simulink model "simulation"  (R2023a)
settings: Solver=ode14x  StartTime=0.0  StopTime=75000.0  FixedStep=optimizerParams.simulinkStepSize  RelTol=1e-3
undefined symbols (not defined in the file or in its folder): ambientTemperatures, batteryParams, gridPricesDayBefore, optimizerParams, panelCurrentParams, panelTemperatureParams, powerDemand, solarIrradiation
libraries: simulink x4, dspsigops x4
settings Model: SimulationMode=accelerator  Creator=jespe  LastModifiedBy=jesperek
settings OptimizationCC: OptimizeBlockIOStorage=off  ReuseModelBlockBuffer=off
settings DebuggingCC: SignalResolutionControl=TryResolveAllWithWarning  SolverPrmCheckMsg=warning  UnderSpecifiedDataTypeMsg=warning  UnnecessaryDatatypeConvMsg=warning  VectorMatrixConversionMsg=warning  SignalLabelMismatchMsg=warning  UnconnectedInputMsg=warning  UnconnectedOutputMsg=warning  UnconnectedLineMsg=warning  SFcnCompatibilityMsg=warning  FrameProcessingCompatibilityMsg=warning  StateNameClashWarn=warning  StrictBusMsg=WarnOnBusTreatedAsVector  NonBusSignalsTreatedAsBus=warning  UnderSpecifiedDimensionMsg=warning
settings RTWCC: GenerateReport=on  BuildConfiguration=Debug  LaunchReport=on
settings CodeAppCC: ForceParamTrailComments=on  MaxIdLength=62  StateflowObjectComments=on  MATLABSourceComments=on

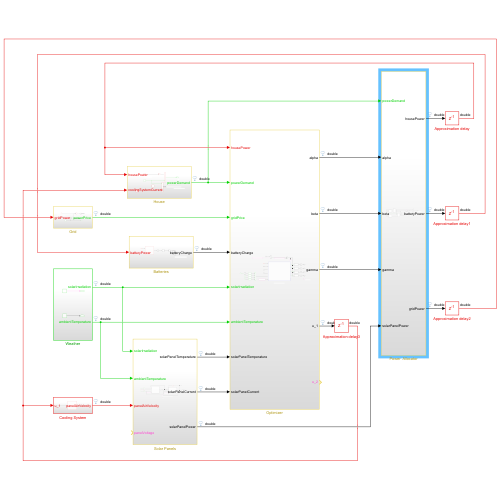
[thumbnail: Simulink's stored preview of the top-level diagram]
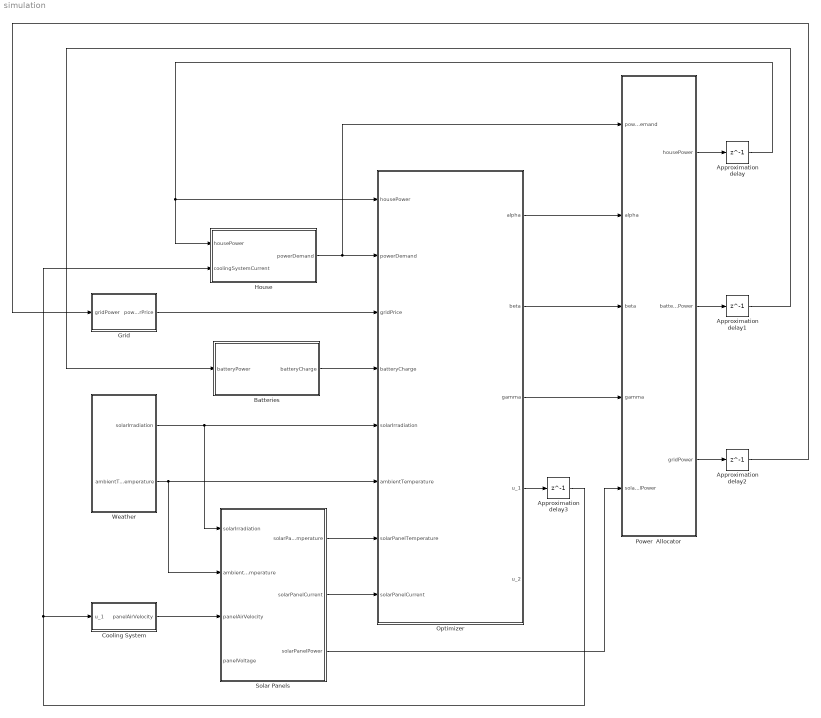
== system simulation ==
  Approximation delay{,1..3} (4 alike) : Delay  DelayLength=1  InitialCondition=0
  Batteries : Subsystem
  Cooling System : Subsystem
  Grid : Subsystem
  House : Subsystem
  Optimizer : Subsystem
  Power  Allocator : Subsystem
  Solar Panels : Subsystem
  Weather : Subsystem
  wires:
  Cooling System/1(panelAirVelocity) -> Solar Panels/3(panelAirVelocity)
  Weather/1(solarIrradiation) -> Solar Panels/1(solarIrradiation), Optimizer/5(solarIrradiation)
  Weather/2(ambientTemperature) -> Optimizer/6(ambientTemperature), Solar Panels/2(ambientTemperature)
  House/1(powerDemand) -> Power  Allocator/1(powerDemand), Optimizer/2(powerDemand)
  Grid/1(powerPrice) -> Optimizer/3(gridPrice)
  Solar Panels/3(solarPanelPower) -> Power  Allocator/5(solarPanelPower)
  Batteries/1(batteryCharge) -> Optimizer/4(batteryCharge)
  Power  Allocator/1(housePower) -> Approximation delay/1
  Power  Allocator/2(batteryPower) -> Approximation delay1/1
  Power  Allocator/3(gridPower) -> Approximation delay2/1
  Optimizer/1(alpha) -> Power  Allocator/2(alpha)
  Optimizer/2(beta) -> Power  Allocator/3(beta)
  Optimizer/3(gamma) -> Power  Allocator/4(gamma)
  Optimizer/4(u_1) -> Approximation delay3/1
  Solar Panels/2(solarPanelCurrent) -> Optimizer/8(solarPanelCurrent)
  Solar Panels/1(solarPanelTemperature) -> Optimizer/7(solarPanelTemperature)
  Approximation delay/1 -> Optimizer/1(housePower), House/1(housePower)
  Approximation delay1/1 -> Batteries/1(batteryPower)
  Approximation delay2/1 -> Grid/1(gridPower)
  Approximation delay3/1 -> Cooling System/1(u_1), House/2(coolingSystemCurrent)

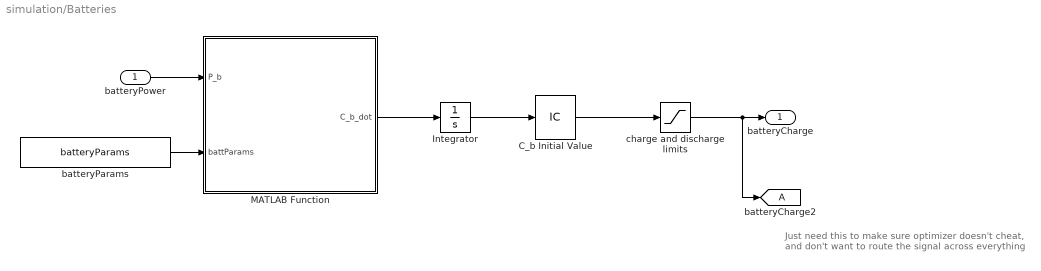
== system simulation/Batteries ==
  note: Just need this to make sure optimizer doesn't cheat,
      | and don't want to route the signal across everything
  batteryPower : Inport
  C_b Initial Value : InitialCondition  Value=0
  Integrator : Integrator
  MATLAB Function : MATLAB Function  TreatAsAtomicUnit=on
  batteryCharge2 : Goto  TagVisibility=global
  batteryParams : Constant  Value=batteryParams  OutDataTypeStr=Bus: battPars
  charge and discharge limits : Saturate  UpperLimit=batteryParams.maxCharge  LowerLimit=0.0
  batteryCharge : Outport
  wires:
  batteryPower/1 -> MATLAB Function/1(P_b)
  batteryParams/1 -> MATLAB Function/2(battParams)
  MATLAB Function/1(C_b_dot) -> Integrator/1
  Integrator/1 -> C_b Initial Value/1
  charge and discharge limits/1 -> batteryCharge/1, batteryCharge2/1
  C_b Initial Value/1 -> charge and discharge limits/1

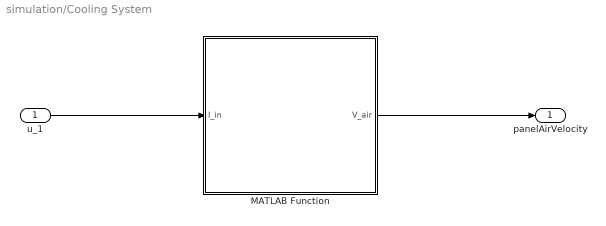
== system simulation/Cooling System ==
  u_1 : Inport
  MATLAB Function : MATLAB Function  TreatAsAtomicUnit=on
  panelAirVelocity : Outport
  wires:
  u_1/1 -> MATLAB Function/1(I_in)
  MATLAB Function/1(V_air) -> panelAirVelocity/1

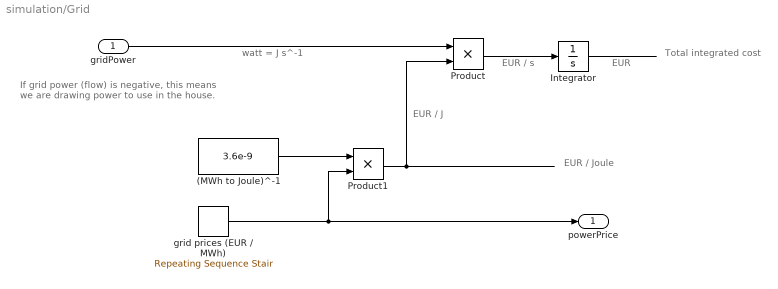
== system simulation/Grid ==
  note: EUR / J
  note: EUR
  note: EUR / s
  note: Total integrated cost
  note: watt = J s^-1
  note: If grid power (flow) is negative, this means
      | we are drawing power to use in the house.
  note: EUR / Joule
  gridPower : Inport
  (MWh to Joule)^-1 : Constant  Value=3.6e-9
  Integrator : Integrator
  Product : Product
  Product1 : Product
  grid prices (EUR / MWh) : simulink/Sources/Repeating Sequence Stair  OutValues=gridPrices  tsamp=1  OutMin=[]  OutMax=[]  OutDataTypeStr=double  OutputDataTypeScalingMode=double  OutDataType=fixdt(0,8)  ConRadixGroup=Best Precision: Vector-wise  OutScaling=2^-12
  powerPrice : Outport
  wires:
  gridPower/1 -> Product/1
  Product1/1 -> Product/2
  (MWh to Joule)^-1/1 -> Product1/1
  grid prices (EUR / MWh)/1 -> powerPrice/1, Product1/2
  Product/1 -> Integrator/1
  Integrator/1 -> ?

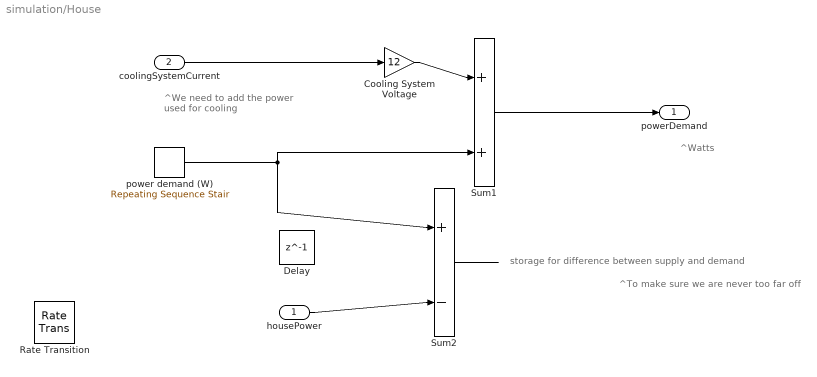
== system simulation/House ==
  note: ^We need to add the power
      |  used for cooling
  note: ^To make sure we are never too far off
  note: storage for difference between supply and demand
  note: ^Watts
  housePower : Inport
  coolingSystemCurrent : Inport  Port=2
  Cooling System Voltage : Gain  Gain=12
  Delay : Delay  DelayLength=1
  Rate Transition : RateTransition
  Sum1 : Sum  Inputs=+|+
  Sum2 : Sum  Inputs=+|-
  power demand (W) : simulink/Sources/Repeating Sequence Stair  OutValues=powerDemand  tsamp=1  OutMin=[]  OutMax=[]  OutDataTypeStr=double  OutputDataTypeScalingMode=double  OutDataType=fixdt(0,8)  ConRadixGroup=Best Precision: Vector-wise  OutScaling=2^-12
  powerDemand : Outport
  wires:
  housePower/1 -> Sum2/2
  Sum2/1 -> ?
  coolingSystemCurrent/1 -> Cooling System Voltage/1
  Cooling System Voltage/1 -> Sum1/1
  power demand (W)/1 -> Sum2/1, Sum1/2
  Sum1/1 -> powerDemand/1

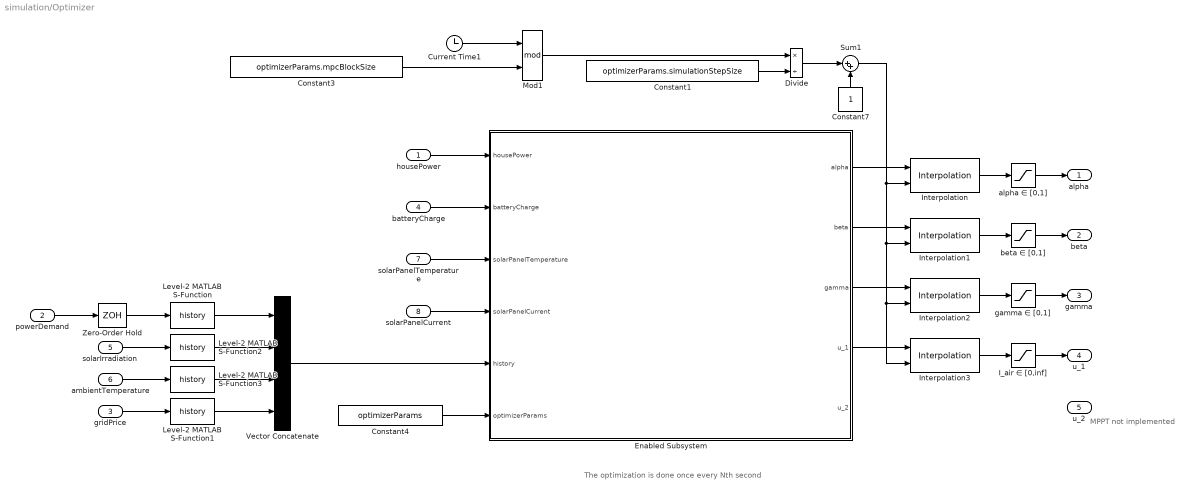
== system simulation/Optimizer ==
  note: The optimization is done once every Nth second
  note: MPPT not implemented
  housePower : Inport
  powerDemand : Inport  Port=2
  gridPrice : Inport  Port=3
  batteryCharge : Inport  Port=4
  solarIrradiation : Inport  Port=5
  ambientTemperature : Inport  Port=6
  solarPanelTemperature : Inport  Port=7
  solarPanelCurrent : Inport  Port=8
  Constant1 : Constant  Value=optimizerParams.simulationStepSize
  Constant3 : Constant  Value=optimizerParams.mpcBlockSize
  Constant4 : Constant  Value=optimizerParams  OutDataTypeStr=Bus: optPars
  Constant7 : Constant
  Current Time1 : Clock
  Divide : Product  Inputs=*/
  "Enabled Subsystem " : Subsystem  TreatAsAtomicUnit=on
  I_air ∈ [0,inf] : Saturate  UpperLimit=99999999  LowerLimit=0
  Interpolation{,1..3} (4 alike) : dspsigops/Interpolation  InterpSource=Input port  InterpPoints=[1.1 4.8 2.67 1.6 3.2]'  InterpMode=Linear  InterpL=3  InterpR=3  InterpAlpha=0.5  InvalidMode=Clip and warn
  Level-2 MATLAB S-Function{,1..3} (4 alike) : M-S-Function  FunctionName=history  Parameters=SECONDS_IN_A_DAY
  Mod1 : Math  Operator=mod  OutputSignalType=real
  Sum1 : Sum  Inputs=|++
  Vector Concatenate : Concatenate  NumInputs=4  Mode=Multidimensional array  ConcatenateDimension=2
  Zero-Order Hold : ZeroOrderHold
  alpha ∈ [0,1] : Saturate  UpperLimit=1  LowerLimit=0
  beta ∈ [0,1] : Saturate  UpperLimit=1  LowerLimit=0
  gamma ∈ [0,1] : Saturate  UpperLimit=1  LowerLimit=0
  alpha : Outport
  beta : Outport  Port=2
  gamma : Outport  Port=3
  u_1 : Outport  Port=4
  u_2 : Outport  Port=5
  wires:
  "Enabled Subsystem "/1(alpha) -> Interpolation/1
  Interpolation/1 -> alpha ∈ [0,1]/1
  "Enabled Subsystem "/2(beta) -> Interpolation1/1
  "Enabled Subsystem "/4(u_1) -> Interpolation3/1
  "Enabled Subsystem "/3(gamma) -> Interpolation2/1
  Interpolation1/1 -> beta ∈ [0,1]/1
  Interpolation2/1 -> gamma ∈ [0,1]/1
  batteryCharge/1 -> "Enabled Subsystem "/2(batteryCharge)
  solarPanelTemperature/1 -> "Enabled Subsystem "/3(solarPanelTemperature)
  Constant4/1 -> "Enabled Subsystem "/6(optimizerParams)
  solarPanelCurrent/1 -> "Enabled Subsystem "/4(solarPanelCurrent)
  Vector Concatenate/1 -> "Enabled Subsystem "/5(history)
  powerDemand/1 -> Zero-Order Hold/1
  gridPrice/1 -> Level-2 MATLAB S-Function1/1
  housePower/1 -> "Enabled Subsystem "/1(housePower)
  solarIrradiation/1 -> Level-2 MATLAB S-Function2/1
  ambientTemperature/1 -> Level-2 MATLAB S-Function3/1
  Level-2 MATLAB S-Function/1 -> Vector Concatenate/1
  Level-2 MATLAB S-Function2/1 -> Vector Concatenate/2
  Level-2 MATLAB S-Function3/1 -> Vector Concatenate/3
  Level-2 MATLAB S-Function1/1 -> Vector Concatenate/4
  Interpolation3/1 -> I_air ∈ [0,inf]/1
  alpha ∈ [0,1]/1 -> alpha/1
  beta ∈ [0,1]/1 -> beta/1
  gamma ∈ [0,1]/1 -> gamma/1
  Constant3/1 -> Mod1/2
  Current Time1/1 -> Mod1/1
  Mod1/1 -> Divide/1
  Constant1/1 -> Divide/2
  Constant7/1 -> Sum1/2
  Divide/1 -> Sum1/1
  Sum1/1 -> Interpolation3/2, Interpolation2/2, Interpolation1/2, Interpolation/2
  I_air ∈ [0,inf]/1 -> u_1/1
  Zero-Order Hold/1 -> Level-2 MATLAB S-Function/1

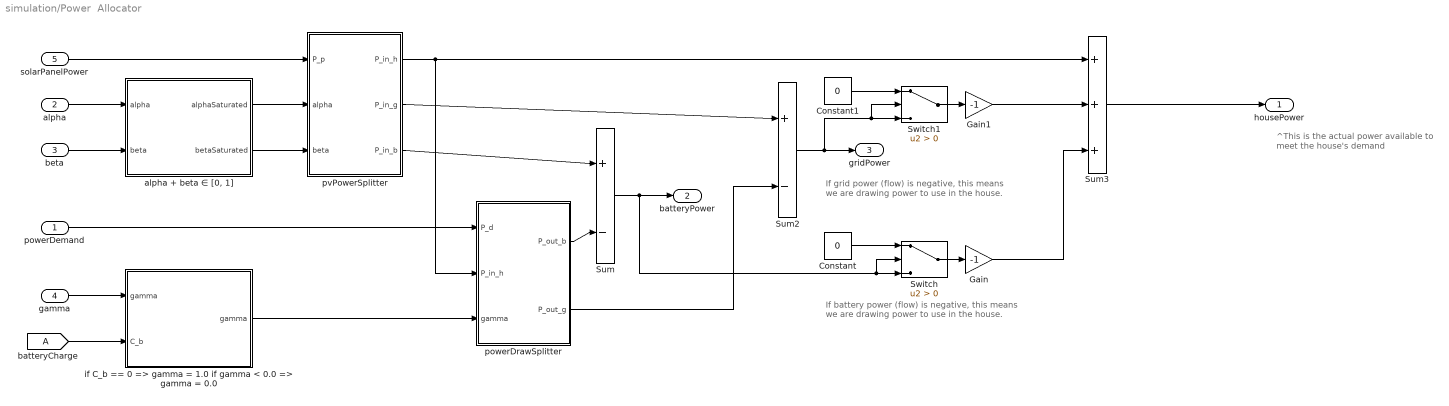
== system simulation/Power  Allocator ==
  note: ^This is the actual power available
      | to meet the house's demand
  note: If battery power (flow) is negative, this means
      | we are drawing power to use in the house.
  note: If grid power (flow) is negative, this means
      | we are drawing power to use in the house.
  powerDemand : Inport
  alpha : Inport  Port=2
  beta : Inport  Port=3
  gamma : Inport  Port=4
  solarPanelPower : Inport  Port=5
  Constant : Constant  Value=0
  Constant1 : Constant  Value=0
  Gain : Gain  Gain=-1
  Gain1 : Gain  Gain=-1
  Sum : Sum  Inputs=+|-
  Sum2 : Sum  Inputs=+|-
  Sum3 : Sum  Inputs=+++
  Switch : Switch  Criteria=u2 > Threshold  SaturateOnIntegerOverflow=off  InputSameDT=off
  Switch1 : Switch  Criteria=u2 > Threshold  SaturateOnIntegerOverflow=off  InputSameDT=off
  "alpha + beta ∈ [0, 1]" : MATLAB Function  TreatAsAtomicUnit=on
  batteryCharge : From  TagVisibility=global
  if C_b == 0 => gamma = 1.0 if gamma < 0.0 => gamma = 0.0 : MATLAB Function  TreatAsAtomicUnit=on
  powerDrawSplitter : MATLAB Function  TreatAsAtomicUnit=on
  pvPowerSplitter : MATLAB Function  TreatAsAtomicUnit=on
  housePower : Outport
  batteryPower : Outport  Port=2
  gridPower : Outport  Port=3
  wires:
  solarPanelPower/1 -> pvPowerSplitter/1(P_p)
  pvPowerSplitter/3(P_in_b) -> Sum/1
  powerDrawSplitter/1(P_out_b) -> Sum/2
  powerDrawSplitter/2(P_out_g) -> Sum2/2
  pvPowerSplitter/2(P_in_g) -> Sum2/1
  Sum2/1 -> Switch1/2, Switch1/3, gridPower/1
  pvPowerSplitter/1(P_in_h) -> powerDrawSplitter/2(P_in_h), Sum3/1
  powerDemand/1 -> powerDrawSplitter/1(P_d)
  Sum/1 -> Switch/2, Switch/3, batteryPower/1
  Switch/1 -> Gain/1
  Constant/1 -> Switch/1
  Gain/1 -> Sum3/3
  Constant1/1 -> Switch1/1
  Switch1/1 -> Gain1/1
  Gain1/1 -> Sum3/2
  alpha/1 -> "alpha + beta ∈ [0, 1]"/1(alpha)
  "alpha + beta ∈ [0, 1]"/1(alphaSaturated) -> pvPowerSplitter/2(alpha)
  beta/1 -> "alpha + beta ∈ [0, 1]"/2(beta)
  "alpha + beta ∈ [0, 1]"/2(betaSaturated) -> pvPowerSplitter/3(beta)
  Sum3/1 -> housePower/1
  gamma/1 -> if C_b == 0 => gamma = 1.0 if gamma < 0.0 => gamma = 0.0/1("gamma ")
  batteryCharge/1 -> if C_b == 0 => gamma = 1.0 if gamma < 0.0 => gamma = 0.0/2(C_b)
  if C_b == 0 => gamma = 1.0 if gamma < 0.0 => gamma = 0.0/1(gamma) -> powerDrawSplitter/3(gamma)

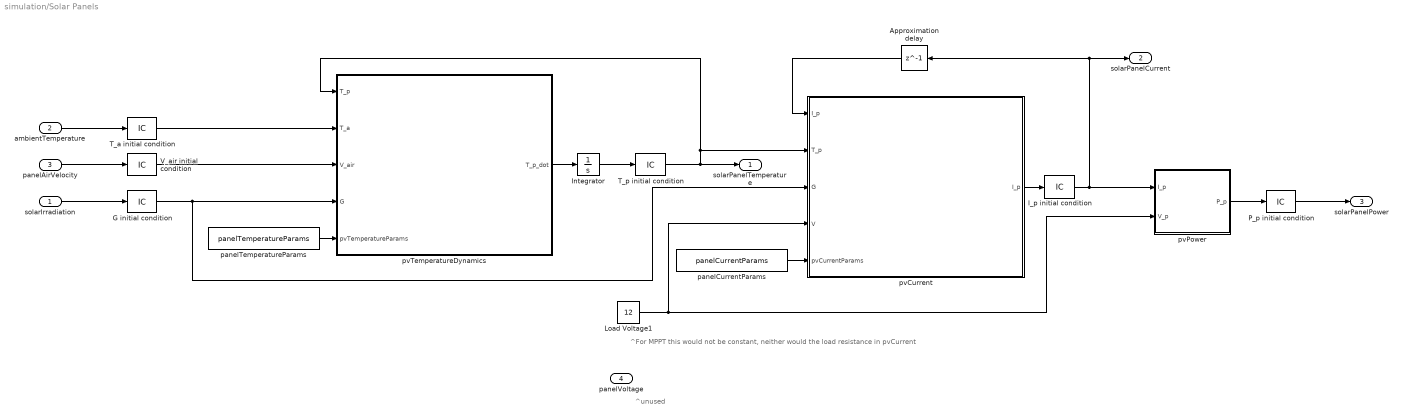
== system simulation/Solar Panels ==
  note: ^unused
  note: ^For MPPT this would not be constant, neither would the load resistance in pvCurrent
  solarIrradiation : Inport
  ambientTemperature : Inport  Port=2
  panelAirVelocity : Inport  Port=3
  panelVoltage : Inport  Port=4
  Approximation delay : Delay  DelayLength=1  InitialCondition=0
  G initial condition : InitialCondition  Value=0
  I_p initial condition : InitialCondition  Value=0
  Integrator : Integrator  InitialCondition=278.65
  Load Voltage1 : Constant  Value=12
  P_p initial condition : InitialCondition  Value=0
  T_a initial condition : InitialCondition  Value=278.65
  T_p initial condition : InitialCondition  Value=278.65
  V_air initial condition : InitialCondition  Value=0
  panelCurrentParams : Constant  Value=panelCurrentParams  OutDataTypeStr=Bus: panCurrPars
  panelTemperatureParams : Constant  Value=panelTemperatureParams  OutDataTypeStr=Bus: panTempPars
  pvCurrent : MATLAB Function  TreatAsAtomicUnit=on
  pvPower : MATLAB Function  TreatAsAtomicUnit=on
  pvTemperatureDynamics : MATLAB Function  TreatAsAtomicUnit=on
  solarPanelTemperature : Outport
  solarPanelCurrent : Outport  Port=2
  solarPanelPower : Outport  Port=3
  wires:
  panelTemperatureParams/1 -> pvTemperatureDynamics/5(pvTemperatureParams)
  panelCurrentParams/1 -> pvCurrent/5(pvCurrentParams)
  pvTemperatureDynamics/1(T_p_dot) -> Integrator/1
  Integrator/1 -> T_p initial condition/1
  pvCurrent/1(I_p) -> I_p initial condition/1
  Approximation delay/1 -> pvCurrent/1("I_p ")
  Load Voltage1/1 -> pvPower/2(V_p), pvCurrent/4(V)
  pvPower/1(P_p) -> P_p initial condition/1
  ambientTemperature/1 -> T_a initial condition/1
  solarIrradiation/1 -> G initial condition/1
  panelAirVelocity/1 -> V_air initial condition/1
  T_a initial condition/1 -> pvTemperatureDynamics/2(T_a)
  V_air initial condition/1 -> pvTemperatureDynamics/3(V_air)
  G initial condition/1 -> pvTemperatureDynamics/4(G), pvCurrent/3(G)
  T_p initial condition/1 -> solarPanelTemperature/1, pvTemperatureDynamics/1(T_p), pvCurrent/2(T_p)
  I_p initial condition/1 -> solarPanelCurrent/1, Approximation delay/1, pvPower/1(I_p)
  P_p initial condition/1 -> solarPanelPower/1

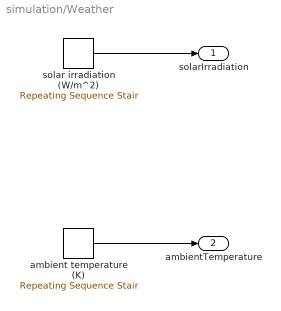
== system simulation/Weather ==
  ambient temperature (K) : simulink/Sources/Repeating Sequence Stair  OutValues=ambientTemperatures  tsamp=1  OutMin=[]  OutMax=[]  OutDataTypeStr=double  OutputDataTypeScalingMode=double  OutDataType=fixdt(0,8)  ConRadixGroup=Best Precision: Vector-wise  OutScaling=2^-12
  solar irradiation (W/m^2) : simulink/Sources/Repeating Sequence Stair  OutValues=solarIrradiation  tsamp=1  OutMin=[]  OutMax=[]  OutDataTypeStr=double  OutputDataTypeScalingMode=double  OutDataType=fixdt(0,8)  ConRadixGroup=Best Precision: Vector-wise  OutScaling=2^-12
  solarIrradiation : Outport
  ambientTemperature : Outport  Port=2
  wires:
  solar irradiation (W/m^2)/1 -> solarIrradiation/1
  ambient temperature (K)/1 -> ambientTemperature/1

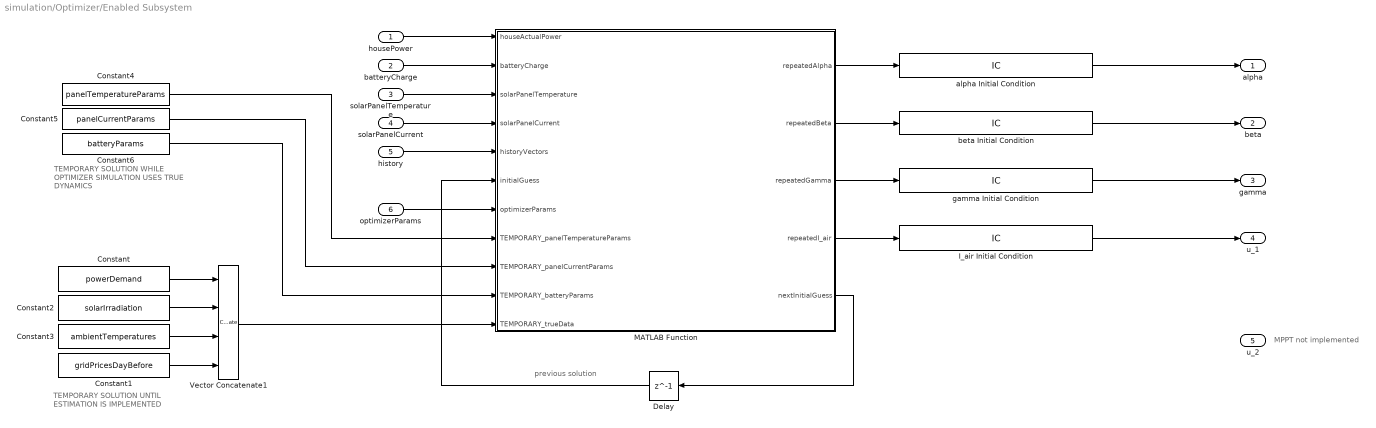
== system simulation/Optimizer/Enabled Subsystem  ==
  note: TEMPORARY SOLUTION UNTIL
      | ESTIMATION IS IMPLEMENTED
  note: MPPT not implemented
  note: previous solution
  note: TEMPORARY SOLUTION WHILE
      | OPTIMIZER SIMULATION USES
      | TRUE DYNAMICS
  housePower : Inport
  batteryCharge : Inport  Port=2
  solarPanelTemperature : Inport  Port=3
  solarPanelCurrent : Inport  Port=4
  history : Inport  Port=5
  optimizerParams : Inport  Port=6
  Constant : Constant  Value=powerDemand
  Constant1 : Constant  Value=gridPricesDayBefore
  Constant2 : Constant  Value=solarIrradiation
  Constant3 : Constant  Value=ambientTemperatures
  Constant4 : Constant  Value=panelTemperatureParams  VectorParams1D=off  OutDataTypeStr=Bus: panTempPars
  Constant5 : Constant  Value=panelCurrentParams  VectorParams1D=off  OutDataTypeStr=Bus: panCurrPars
  Constant6 : Constant  Value=batteryParams  VectorParams1D=off  OutDataTypeStr=Bus: battPars  LockScale=on
  Delay : Delay  DelayLength=1  InitialCondition=0.26*ones(optimizerParams.numControlInputs*optimizerParams.controlVariableHorizon, 1)
  I_air Initial Condition : InitialCondition  Value=zeros(optimizerParams.optimizationHorizon, 1)
  MATLAB Function : MATLAB Function  TreatAsAtomicUnit=on  SystemSampleTime=optimizerParams.mpcBlockSize
      settings: MinAlgLoopOccurrences=on
  Vector Concatenate1 : Concatenate  NumInputs=4  Mode=Multidimensional array  ConcatenateDimension=2
  alpha Initial Condition : InitialCondition  Value=0.26*ones(optimizerParams.optimizationHorizon, 1)
  beta Initial Condition : InitialCondition  Value=0.25*ones(optimizerParams.optimizationHorizon, 1)
  gamma Initial Condition : InitialCondition  Value=ones(optimizerParams.optimizationHorizon, 1)
  alpha : Outport
  beta : Outport  Port=2
  gamma : Outport  Port=3
  u_1 : Outport  Port=4
  u_2 : Outport  Port=5
  wires:
  Delay/1 -> MATLAB Function/6(initialGuess)
  batteryCharge/1 -> MATLAB Function/2(batteryCharge)
  history/1 -> MATLAB Function/5(historyVectors)
  solarPanelTemperature/1 -> MATLAB Function/3(solarPanelTemperature)
  solarPanelCurrent/1 -> MATLAB Function/4(solarPanelCurrent)
  optimizerParams/1 -> MATLAB Function/7(optimizerParams)
  Constant/1 -> Vector Concatenate1/1
  Constant2/1 -> Vector Concatenate1/2
  Constant3/1 -> Vector Concatenate1/3
  Constant1/1 -> Vector Concatenate1/4
  Vector Concatenate1/1 -> MATLAB Function/11(TEMPORARY_trueData)
  housePower/1 -> MATLAB Function/1(houseActualPower)
  Constant4/1 -> MATLAB Function/8(TEMPORARY_panelTemperatureParams)
  Constant5/1 -> MATLAB Function/9(TEMPORARY_panelCurrentParams)
  Constant6/1 -> MATLAB Function/10(TEMPORARY_batteryParams)
  MATLAB Function/1(repeatedAlpha) -> alpha Initial Condition/1
  MATLAB Function/2(repeatedBeta) -> beta Initial Condition/1
  MATLAB Function/3(repeatedGamma) -> gamma Initial Condition/1
  MATLAB Function/4(repeatedI_air) -> I_air Initial Condition/1
  I_air Initial Condition/1 -> u_1/1
  gamma Initial Condition/1 -> gamma/1
  beta Initial Condition/1 -> beta/1
  alpha Initial Condition/1 -> alpha/1
  MATLAB Function/5(nextInitialGuess) -> Delay/1

== matlab function simulation/Power  Allocator/alpha + beta ∈ [0, 1] ==
  data: alpha input; alphaSaturated output; beta input; betaSaturated output
function [alphaSaturated, betaSaturated] = fcn(alpha, beta)
% We need to make sure the actual control inputs don't violate constraints
    if (alpha + beta > 1.0)
        diff = (alpha + beta) - 1;
        alphaSaturated = alpha - 0.5*diff;
        betaSaturated  = beta - 0.5*diff;
    else
        alphaSaturated = alpha;
        betaSaturated = beta;
    end
end

== matlab function simulation/Optimizer/Enabled Subsystem /MATLAB Function ==
  data: houseActualPower input double; repeatedAlpha output double size=[optimizerParams.optimizationHorizon, 1]; repeatedBeta output double size=[optimizerParams.optimizationHorizon, 1]; repeatedGamma output double size=[optimizerParams.optimizationHorizon, 1]; repeatedI_air output double size=[optimizerParams.optimizationHorizon, 1]; batteryCharge input double; solarPanelTemperature input double; solarPanelCurrent input double; historyVectors input double; initialGuess input double size=[optimizerParams.numControlInputs*optimizerParams.controlVariableHorizon, 1]; optimizerParams input Bus: optPars; TEMPORARY_panelTemperatureParams input Bus: panTempPars; TEMPORARY_panelCurrentParams input Bus: panCurrPars; TEMPORARY_batteryParams input Bus: battPars; TEMPORARY_trueData input double; nextInitialGuess output double size=[optimizerParams.numControlInputs*optimizerParams.controlVariableHorizon, 1]
function [repeatedAlpha, repeatedBeta, repeatedGamma, repeatedI_air, nextInitialGuess] = optimizer(...
                                                 houseActualPower,...
                                                 batteryCharge,...
                                                 solarPanelTemperature,...
                                                 solarPanelCurrent,...
                                                 historyVectors,...
                                                 initialGuess,...
                                                 optimizerParams,...
                                                 TEMPORARY_panelTemperatureParams,...
                                                 TEMPORARY_panelCurrentParams,...
                                                 TEMPORARY_batteryParams,...
                                                 TEMPORARY_trueData)
    
    persistent N K C singleControlInputLength justSomeOnes;
    if isempty(N); N = optimizerParams.optimizationHorizon; end
    if isempty(K); K = optimizerParams.controlVariableHorizon; end
    if isempty(C); C = optimizerParams.numControlInputs; end
    if isempty(singleControlInputLength); singleControlInputLength = N / K; end
    if isempty(justSomeOnes); justSomeOnes = ones([singleControlInputLength, 1]); end

    coder.extrinsic("Optimizer") % debugging with codegen turned out to be too much of a pain in the ass
    [alpha, beta, gamma, I_air] = Optimizer(...
                                            houseActualPower,...
                                            batteryCharge,...
                                            solarPanelTemperature,...
                                            solarPanelCurrent,...
                                            historyVectors,...
                                            initialGuess,...
                                            optimizerParams,...
                                            TEMPORARY_panelTemperatureParams,...
                                            TEMPORARY_panelCurrentParams,...
                                            TEMPORARY_batteryParams,...
                                            TEMPORARY_trueData...
                                           );

    repeatedAlpha   = kron(alpha, justSomeOnes);
    repeatedBeta    = kron(beta,  justSomeOnes);
    repeatedGamma   = kron(gamma, justSomeOnes); 
    repeatedI_air   = kron(I_air, justSomeOnes);  

    nextInitialGuess = [alpha; beta; gamma; I_air];
end
% Remember that changes to the inputs or outputs 
% of the actual optimizer() must also be reflected here.

== matlab function simulation/Power  Allocator/if C_b == 0 => gamma = 1.0 if gamma < 0.0 => gamma = 0.0 ==
  data: gamma input; gamma output; C_b input
function gamma  = fcn(gamma, C_b)
% We need to make sure the actual control inputs don't violate constraints
    if C_b <= 0.0
        gamma = 1.0;
    end
    if gamma < 0.0
        gamma = 0.0;
    end
end

== matlab function simulation/Solar Panels/pvCurrent ==
  data: I_p input; T_p input; G input; V input; I_p output; pvCurrentParams input
function I_p = pvCurrent(I_p, T_p, G, V, pvCurrentParams)
    I_p = pvCurrent(I_p, T_p, G, V, pvCurrentParams);
end
% Remember that changes to the inputs or outputs 
% of the actual pvCurrentDynamics() must also be reflected here.

== matlab function simulation/Solar Panels/pvTemperatureDynamics ==
  data: T_p_dot output; T_p input; T_a input; V_air input; G input; pvTemperatureParams input
function T_p_dot = pvTemperatureDynamics(T_p, T_a, V_air, G, pvTemperatureParams)
    T_p_dot = pvTemperatureDynamics(T_p, T_a, V_air, G, pvTemperatureParams);
end
% Remember that changes to the inputs or outputs 
% of the actual pvTemperatureDynamics() must also be reflected here.

== matlab function simulation/Solar Panels/pvPower ==
  data: I_p input; V_p input; P_p output
function P_p = pvPower(I_p, V_p)
    P_p = pvPower(I_p, V_p);
end
% Remember that changes to the inputs or outputs 
% of the actual pvPower() must also be reflected here.

== matlab function simulation/Batteries/MATLAB Function ==
  data: P_b input; C_b_dot output; battParams input
function C_b_dot = batteryDynamics(P_b, battParams)
    C_b_dot = batteryDynamics(P_b, battParams);
end

== matlab function simulation/Power  Allocator/powerDrawSplitter ==
  data: P_out_b output; P_d input; P_in_h input; P_out_g output; gamma input
function [P_out_b, P_out_g] = powerDrawSplitter(P_d, P_in_h, gamma)
    [P_out_b, P_out_g] = powerDrawSplitter(P_d, P_in_h, gamma);
end
% Remember that changes to the inputs or outputs 
% of the actual powerDrawSplitter() must also be reflected here.

== matlab function simulation/Power  Allocator/pvPowerSplitter ==
  data: P_p input; alpha input; P_in_h output; beta input; P_in_g output; P_in_b output
function [P_in_h, P_in_g, P_in_b] = pvPowerSplitter(P_p, alpha, beta)
    [P_in_h, P_in_g, P_in_b] = pvPowerSplitter(P_p, alpha, beta);
end
% Remember that changes to the inputs or outputs 
% of the actual pvPowerSplitter() must also be reflected here.

== matlab function simulation/Cooling System/MATLAB Function ==
  data: I_in input; V_air output
function V_air = airCooler(I_in)
    V_air = airCooler(I_in);
end
